simulink model "Flightsim_attitudecontrolled"  (R2024b)
settings: Solver=ode4  StartTime=0.0  StopTime=18  FixedStep=0.01  MaxStep=0.005  MinStep=0.005  RelTol=1e-6  AbsTol=1e-8
values from neighbouring files (symbols this model uses):
  f = fn{i}    [LandingAnalysis.m]    (also in PerformanceAnalysis.m = @(a) obj.lift_residual(alt,V,M,rho,L_target,a,throttle); TakeoffAnalysis.m)
undefined symbols (not defined in the file or in its folder): Earth, u_hover10, WGS84
libraries: simulink_extras x2, aerolibfltsims x2, instrumentlib x2, shared6dof x1, slpidlib x1, aerolibtransform2 x1
settings Model: Creator=naman  LastModifiedBy=naman
settings DataIOCC: OutputSaveName=out

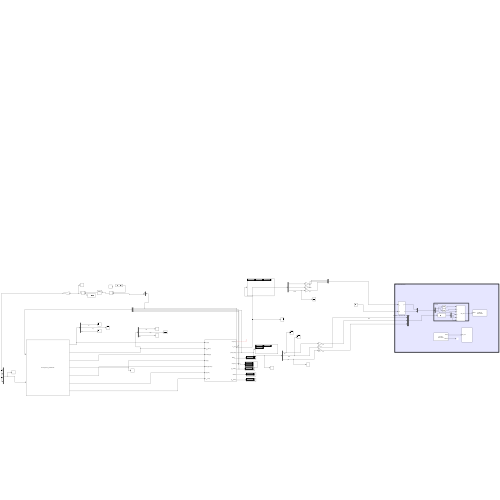
[thumbnail: Simulink's stored preview of the top-level diagram]
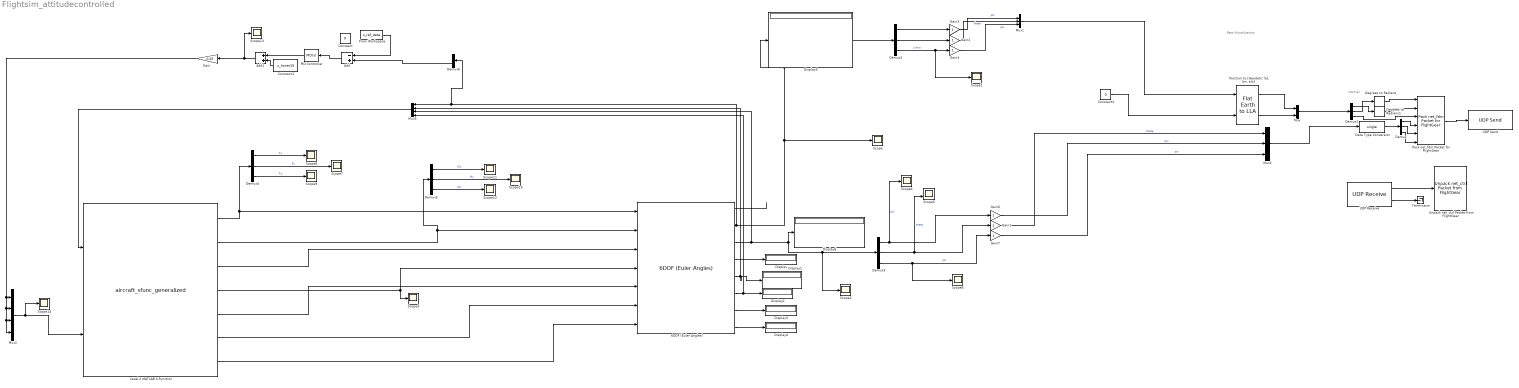
== system Flightsim_attitudecontrolled ==
  note: New Visualization
  note: Inertial
  6DOF (Euler Angles) : shared6dof/6DOF (Euler Angles)  units=Metric (MKS)  mtype=Custom Variable  rep=Euler Angles  xme_0=Initialpos  Vm_0=InitialVel  eul_0=InitialOri  pm_0=InitialRot  mass_0=mass  mass_e=0.5  mass_f=2.0  inertia=[0.02 0 0;0 0.02 0;0 0 0.04]  inertia_e=eye(3)  inertia_f=2*eye(3)  k_quat=1.0  vre_flag=on  abi_flag=off  aMode=0  xme_statename=''  Vm_statename=''  eul_statename=''  quat_statename=''  pm_statename=''  mass_statename=''
  Add : Sum  Inputs=-+
  Add1 : Sum
  Constant : Constant  Value=0
  Constant1 : Constant  Value=u_hover10
  Constant2 : Constant  Value=0
  Data Type Conversion : DataTypeConversion  OutDataTypeStr=single  SaturateOnIntegerOverflow=off  RndMeth=Floor
  Degrees to Radians : simulink_extras/Transformations/Degrees to Radians
  Degrees to Radians1 : simulink_extras/Transformations/Degrees to Radians
  Demux{,1..6} (7 alike) : Demux  Outputs=3
  Display{,1..6} (7 alike) : Display
  From Workspace : FromWorkspace  VariableName=z_ref_data
  Gain : Gain  Gain=0.25
  Gain{1..4,6..7} (6 alike) : Gain
  Level-2 MATLAB S-Function : M-S-Function  FunctionName=aircraft_sfunc_generalized
  Mux : Mux  Inputs=2
  Mux1 : Mux  Inputs=3
  Mux2 : Mux
  Mux3 : Mux  Inputs=3
  Mux5 : Mux
  PID Controller : slpidlib/PID Controller  Controller=PID  Form=Parallel  TimeDomain=Continuous-time  UseExternalTs=off  SampleTime=-1  IntegratorMethod=Forward Euler  FilterMethod=Forward Euler  ControllerParametersSource=internal  P=2  I=0.1  UseKiTs=off  D=3  UseExternalDerivativeSource=off  N=20  UseFilter=on  TunerSelectOption=Transfer Function Based (PID Tuner App)  InitialConditionSource=internal  InitialConditionForIntegrator=0  InitialConditionForFilter=0  DifferentiatorICPrevScaledInput=0  ExternalReset=none  TrackingMode=off  Kt=1  LimitOutput=off  SatLimitsSource=internal  UpperSaturationLimit=inf  LowerSaturationLimit=-inf  LinearizeAsGain=on  AntiWindupMode=none  Kb=1  LimitIntegrator=off  UpperIntegratorSaturationLimit=inf  LowerIntegratorSaturationLimit=-inf  POutMin=[]  POutMax=[]  IOutMin=[]  IOutMax=[]  DOutMin=[]  DOutMax=[]  NOutMin=[]  NOutMax=[]  SumOutMin=[]  SumOutMax=[]  SaturationOutMin=[]  SaturationOutMax=[]  PParamMin=[]  PParamMax=[]  IParamMin=[]  IParamMax=[]  DParamMin=[]  DParamMax=[]  NParamMin=[]  NParamMax=[]  KbParamMin=[]  KbParamMax=[]  KtParamMin=[]  KtParamMax=[]  KbOutMin=[]  KbOutMax=[]  KtOutMin=[]  KtOutMax=[]  IntegratorOutMin=[]  IntegratorOutMax=[]  FilterOutMin=[]  FilterOutMax=[]  SumI1OutMin=[]  SumI1OutMax=[]  SumI2OutMin=[]  SumI2OutMax=[]  SumI3OutMin=[]  SumI3OutMax=[]  SumI4OutMin=[]  SumI4OutMax=[]  SumDOutMin=[]  SumDOutMax=[]  DifferentiatorOutMin=[]  DifferentiatorOutMax=[]  FilterDiffOutCoefMin=[]  FilterDiffOutCoefMax=[]  ReciprocalOutMin=[]  ReciprocalOutMax=[]  SumDenOutMin=[]  SumDenOutMax=[]  SumNumOutMin=[]  SumNumOutMax=[]  DivideOutMin=[]  DivideOutMax=[]  UdiffTsProdOutMin=[]  UdiffTsProdOutMax=[]  NTsProdOutMin=[]  NTsProdOutMax=[]  UintegralTsProdOutMin=[]  UintegralTsProdOutMax=[]  UngainTsProdOutMin=[]  UngainTsProdOutMax=[]  ClampingZeroOutDataTypeStr=Inherit: Inherit via back propagation  ClampingZeroOutMin=[]  ClampingZeroOutMax=[]  FilterDenConstantOutDataTypeStr=Inherit: Inherit via back propagation  FilterDenConstantOutMin=[]  FilterDenConstantOutMax=[]  PCopyOutDataTypeStr=Inherit: Inherit via back propagation  PCopyOutMin=[]  PCopyOutMax=[]  NCopyOutDataTypeStr=Inherit: Inherit via back propagation  NCopyOutMin=[]  NCopyOutMax=[]  IntegratorContinuousStateAttributes=''  IntegratorStateMustResolveToSignalObject=off  IntegratorRTWStateStorageClass=Auto  FilterContinuousStateAttributes=''  FilterStateMustResolveToSignalObject=off  FilterRTWStateStorageClass=Auto  ParallelPVariant=InternalParameters  IdealPVariant=Disabled  IVariant=InternalParameters  DVariant=InternalParameters  IntegratorVariant=Continuous  SatVariant=Disabled  AWVariant=Passthrough  PCopyVariant=Disabled  TRVariant=Disabled  FdbkBlocksVariant=Forward  IdealPFdbkVariant=Disabled  SatFdbkVariant=Disabled  DerivativeFilterVariant=ContFilter  NVariant=InternalParameters  NCopyVariant=Disabled  FilterICVariant=InternalICsFilter  IntegratorICVariant=InternalICs  ExternalResetVariant=Disabled  TRSumVariant=Passthrough  SumFdbkVariant=Disabled  SumVariant=Sum_PID  TsampFilterVariant=InternalTs  TsampNgainVariant=Passthrough  TsampIntegralVariant=Disabled_SignalSpec  ExternalSaturationOutDataTypeStr=Inherit: Same as second input  DerivativeSourceVariant=ErrorSignal  PreIntVariant=InternalPreInt
  Pack net_fdm Packet for FlightGear : aerolibfltsims/Pack net_fdm Packet for FlightGear  FlightGearVersion=v2019.1  ShowPositionAttitudeInputs=on  ShowVelocityAccelerationInputs=off  ShowControlSurfacePositionInputs=off  ShowEngineFuelInputs=off  ShowLandingGearInputs=off  ShowEnvironmentInputs=off  SampleTime=-1  packetVersion=24
  "Position to [Geodetic lat, lon, alti]" : aerolibtransform2/Flat Earth to LLA  units=Metric (MKS)  ptype=Earth (WGS84)  F=1/298.257223563  R=6378137  refPosPort=off  LL0=[37.210265015306916, -80.41446644179189]  psi=0
  Scope{,1..4,6..14} (14 alike) : Scope
  Scope5 : Scope  NumInputPorts=2
  Terminator : Terminator
  UDP Receive : instrumentlib/UDP Receive  LocalAddress=127.0.0.1  LocalPort=50001  EnablePortSharing=off  Host=localhost  Port=65343  GetLatestData=on  DataSize=[ 1, 744 ]  DataType=uint8  ASCIIFormatting=%f,  Terminator=LF  CustomTerminator=10  ByteOrder=little-endian  EnableBlockingMode=off  Timeout=10  SampleTime=0.2  SimulateUsing=Interpreted execution
  UDP Send : instrumentlib/UDP Send  Host=localhost  Port=50000  LocalAddress=127.0.0.1  LocalPort=-1  EnablePortSharing=on  OutputDatagramPacketSize=4096  ByteOrder=big-endian  EnableBlockingMode=on  SimulateUsing=Interpreted execution
  Unpack net_ctrl Packet from FlightGear : aerolibfltsims/Unpack net_ctrl Packet from FlightGear  FlightGearVersion=v2019.1  ShowControlSurfacePositionOutputs=off  ShowEngineFuelOutputs=off  ShowLandingGearOutputs=off  ShowAvionicOutputs=off  ShowEnvironmentOutputs=off  SampleTime=-1  packetVersion=27
  wires:
  UDP Receive/1 -> Unpack net_ctrl Packet from FlightGear/1
  "Position to [Geodetic lat, lon, alti]"/2 -> Mux/2
  Demux/3 -> Pack net_fdm Packet for FlightGear/6
  Gain1/1 -> Mux3/1  "theta"
  Demux1/2 -> Degrees to Radians/1
  Degrees to Radians1/1 -> Pack net_fdm Packet for FlightGear/2
  Gain6/1 -> Mux3/2  "phi"
  Data Type Conversion/1 -> Demux/1
  Demux/1 -> Pack net_fdm Packet for FlightGear/4
  Demux/2 -> Pack net_fdm Packet for FlightGear/5
  UDP Receive/2 -> Terminator/1
  "Position to [Geodetic lat, lon, alti]"/1 -> Mux/1
  Demux1/3 -> Pack net_fdm Packet for FlightGear/3
  Gain7/1 -> Mux3/3  "psi"
  Pack net_fdm Packet for FlightGear/1 -> UDP Send/1
  Degrees to Radians/1 -> Pack net_fdm Packet for FlightGear/1
  Demux1/1 -> Degrees to Radians1/1
  Mux/1 -> Demux1/1
  6DOF (Euler Angles)/4 -> Display/1
  6DOF (Euler Angles)/3 -> Mux5/3, Display6/1, Scope2/1, Demux3/1
  Demux3/1 -> Scope4/1, Gain6/1  "phi"
  Demux3/3 -> Scope6/1, Gain7/1  "psi"
  6DOF (Euler Angles)/5 -> Mux5/2, Display1/1
  6DOF (Euler Angles)/6 -> Mux5/4, Display2/1
  6DOF (Euler Angles)/7 -> Display3/1
  6DOF (Euler Angles)/8 -> Display4/1
  Demux2/1 -> Gain3/1
  Demux2/3 -> Scope1/1, Gain4/1  "z axis"
  Demux2/2 -> Gain2/1
  Gain4/1 -> Mux1/3  "psi"
  Gain3/1 -> Mux1/1  "phi"
  Gain2/1 -> Mux1/2  "theta"
  Mux1/1 -> "Position to [Geodetic lat, lon, alti]"/1
  Constant2/1 -> "Position to [Geodetic lat, lon, alti]"/2
  6DOF (Euler Angles)/1 -> ?
  6DOF (Euler Angles)/2 -> Demux6/1, Mux5/1, Scope/1, Demux2/1, Display5/1
  Mux5/1 -> Level-2 MATLAB S-Function/1
  Level-2 MATLAB S-Function/3 -> 6DOF (Euler Angles)/3
  Level-2 MATLAB S-Function/4 -> Scope3/1, 6DOF (Euler Angles)/4
  Demux3/2 -> Scope5/2, Gain1/1  "theta"
  Demux4/1 -> Scope8/1  "Fx"
  Demux4/2 -> Scope7/1  "Fy"
  Level-2 MATLAB S-Function/1 -> Demux4/1, 6DOF (Euler Angles)/1
  Demux4/3 -> Scope9/1  "Fz"
  Demux5/3 -> Scope12/1  "Mz"
  Demux5/2 -> Scope10/1  "My"
  Level-2 MATLAB S-Function/2 -> Demux5/1, 6DOF (Euler Angles)/2
  Demux5/1 -> Scope11/1  "Mx"
  Level-2 MATLAB S-Function/5 -> 6DOF (Euler Angles)/5
  Level-2 MATLAB S-Function/6 -> 6DOF (Euler Angles)/6
  Mux3/1 -> Data Type Conversion/1
  Level-2 MATLAB S-Function/7 -> 6DOF (Euler Angles)/7
  From Workspace/1 -> Add/1
  Add/1 -> PID Controller/1
  PID Controller/1 -> Add1/1
  Constant1/1 -> Add1/2
  Add1/1 -> Scope13/1, Gain/1
  Mux2/1 -> Scope14/1, Level-2 MATLAB S-Function/2
  Demux6/3 -> Add/2
  Gain/1 -> Mux2/4, Mux2/3, Mux2/2, Mux2/1
